simulink model "mcb_c2000_open_loop_control_host_model"  (R2021b)
settings: Solver=FixedStepDiscrete  StartTime=0.0  StopTime=inf  RelTol=1e-3  EnableMultiTasking=on
InitFcn:
  | if( strcmp(get_param([gcs '/Serial Communication/HW_Selected'], 'Value'), '0'))
  |       set_param([gcs '/Host Serial Setup'], 'baudRateA', '1.5e6');
  | elseif( strcmp(get_param([gcs '/Serial Communication/HW_Selected'], 'Value'), '1'))
  |       set_param([gcs '/Host Serial Setup'], 'baudRateA', '3.75e6');
  | elseif( strcmp(get_param([gcs '/Serial Communication/HW_Selected'], 'Value'), '2'))
  |       set_param([gcs '/Host Serial Setup'], 'baudRateA', '6.25e6');
  | end
values from neighbouring files (symbols this model uses):
  Ts = 5e-8    (= 5e-08)    [DCDC_Buck_Param.m]    (also in mcb_c2000_open_loop_control_data.m = T_pwm; mcb_c2000_pmsm_offset_data.m = T_pwm; mcb_pmsm_foc_dual_f28379d_data.m = 5e-05; mcb_pmsm_foc_dual_f28379d_datascript.m = 5e-05)
libraries: mcbhostblockslib x3, demo_controls x1
PreSaveFcn:
  | if( strcmp(get_param([gcs '/Serial Communication/HW_Selected'], 'Value'), '0'))
  |       set_param([gcs '/Host Serial Setup'], 'baudRateA', '1.5e6');
  | elseif( strcmp(get_param([gcs '/Serial Communication/HW_Selected'], 'Value'), '1'))
  |       set_param([gcs '/Host Serial Setup'], 'baudRateA', '3.75e6');
  | elseif( strcmp(get_param([gcs '/Serial Communication/HW_Selected'], 'Value'), '2'))
  |       set_param([gcs '/Host Serial Setup'], 'baudRateA', '6.25e6');
  | end
settings Model: Creator=The MathWorks, Inc.  LastModifiedBy=The MathWorks, Inc.
settings SolverCC: AlgebraicLoopSolver=TrustRegion
settings DataIOCC: LimitDataPoints=on  SaveFormat=Array  ReturnWorkspaceOutputs=off
settings OptimizationCC: LifeSpan=1  EfficientTunableParamExpr=on
settings DebuggingCC: UnderspecifiedInitializationDetection=Classic  MergeDetectMultiDrivingBlocksExec=none  SolverPrmCheckMsg=warning  ParameterPrecisionLossMsg=none  AllowSymbolicDim=off  PregeneratedLibrarySubsystemCodeDiagnostic=none  SFUnexpectedBacktrackingDiag=warning  SFNoUnconditionalDefaultTransitionDiag=warning  SFExecutionAtInitializationDiag=none  SFMachineParentedDataDiag=warning  ArithmeticOperatorsInVariantConditions=warning
settings HardwareCC: ProdBitPerPointer=32  ProdLargestAtomicFloat=None  ProdIntDivRoundTo=Undefined  ProdEndianess=Unspecified  ProdWordSize=32  ProdHWDeviceType=32-bit Generic
settings ModelReferenceCC: PropagateSignalLabelsOutOfModel=off
settings SFSimCC: SimUseLocalCustomCode=off  MATLABDynamicMemAlloc=off
settings RTWCC: Description=Real-Time Workshop Embedded Coder  SystemTargetFile=ert.tlc  TemplateMakefile=ert_default_tmf  GenerateReport=on  RTWUseLocalCustomCode=off  IncludeHyperlinkInReport=on  LaunchReport=on  GenerateTraceInfo=on  GenerateTraceReport=on  GenerateTraceReportSl=on  GenerateTraceReportSf=on  GenerateTraceReportEml=on
settings CodeAppCC: IgnoreCustomStorageClasses=off  StateflowObjectComments=on  InternalIdentifier=Classic
settings ERTTargetCC: MultiwordLength=2048  GenerateSampleERTMain=on  ERTCustomFileTemplate=example_file_process.tlc  ConvertIfToSwitch=off  SuppressUnreachableDefaultCases=off
settings ConfigComp: CovMetricSettings=dw  CovSaveCumulativeToWorkspaceVar=on  CovSaveSingleToWorkspaceVar=on  CovExternalEMLEnable=off  CovSFcnEnable=off

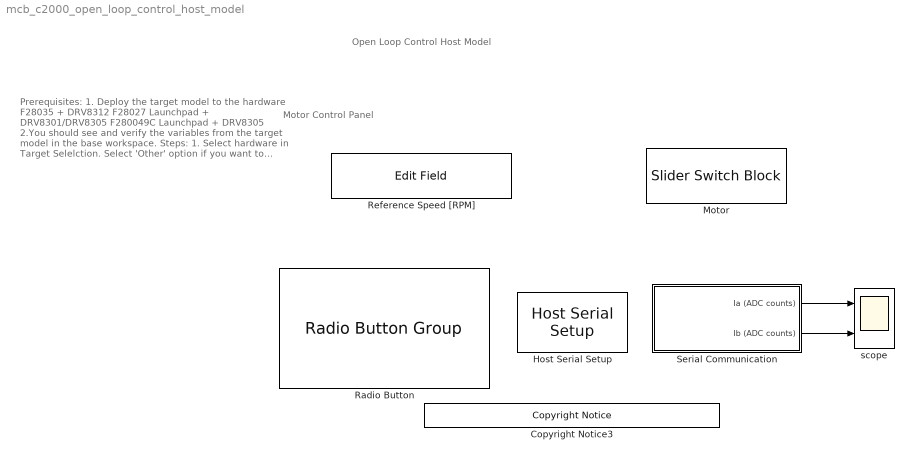
== system mcb_c2000_open_loop_control_host_model ==
  note: Open Loop Control Host Model
  note: Motor Control Panel
  note: Prerequisites:
      | 1. Deploy the target model to the hardware
      | F28035 + DRV8312
      | F28027 Launchpad + DRV8301/DRV8305
      | F280049C Launchpad + DRV8305
      | 2.You should see and verify the variables
      | from the target model in the base
      | workspace.
      |
      | Steps:
      | 1. Select hardware in Target Selelction.
      | Select 'Other' option if you want to manually set
      | the baud rate in 'Host Serial Setup' block.
      | 2. Select the serial port in ' Serial 1 ' tab of ' Host
      | Serial Setup ' block.
      | 3. Use ' Motor Start / Stop ' switch to control the
      | motor.
      | 4. Enter speed request in RPM using 'Reference
      | Speed' edit box. Limit the reference speed to
      | half of the rated speed.
      | 5. Observe the ADC counts for phase current
      | measurent in Scope.
  Copyright Notice3 : demo_controls/Copyright Notice  year=2021  prod=tic2000
      settings: SourceProductBaseCode=ME
  Host Serial Setup : mcbhostblockslib/Host Serial Setup  Priority=-99  comPortSer1='Please_select_a_port'  baudRateA=1.5e6  charLenA=8  stopBitA=1  parityA=none  timeoutA=2  ByteOrderA=LittleEndian  comPortSer2='Please_select_a_port'  baudRateB=115200  charLenB=8  stopBitB=1  parityB=none  timeoutB=1.0  ByteOrderB=LittleEndian  comPortSer3='Please_select_a_port'  baudRateC=115200  charLenC=8  stopBitC=1  parityC=none  timeoutC=1.0  ByteOrderC=LittleEndian  comPortSer4='Please_select_a_port'  baudRateD=115200  charLenD=8  stopBitD=1  parityD=none  timeoutD=1.0  ByteOrderD=LittleEndian
      settings: SourceProductBaseCode=MT
  Motor : SliderSwitchBlock  LabelPosition=Hide
      settings: Values={{'Stop', 'Start'}, [0 1]}
  Radio Button : RadioButtonGroup  LabelPosition=Hide  SelectedLabel=TI F28035  ButtonGroupName=Target Selection
      settings: Values={{'TI F28035', 'TI F28027', 'TI F280049C', 'Other'}, [0 1 2 3]}
  Reference Speed [RPM] : EditField  LabelPosition=Hide  ShowInitialText=on  Alignment=Center
  Serial Communication : Subsystem
  scope : Scope  NumInputPorts=2
  wires:
  Serial Communication/1(Ia (ADC counts)) -> scope/1
  Serial Communication/2(Ib (ADC counts)) -> scope/2

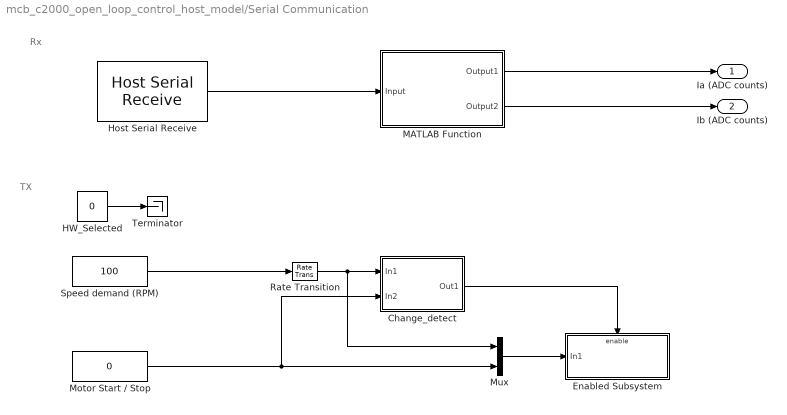
== system mcb_c2000_open_loop_control_host_model/Serial Communication ==
  note: TX
  note: Rx
  Change_detect : Subsystem
  Enabled Subsystem : Subsystem  TreatAsAtomicUnit=on
  HW_Selected : Constant  Value=0  OutDataTypeStr=uint8
  Host Serial Receive : mcbhostblockslib/Host Serial Receive  serialCon=Serial 1  dataHead='SS'  dataTail='EE'  dataType=uint16  dataDim=[600 2]  initValue=0  errOption=Output the last received value  errValue=0  sampleTime=600 * Ts  outputStatus=off  blockingMode=on
      settings: SourceProductBaseCode=MT
  MATLAB Function : MATLAB Function  TreatAsAtomicUnit=on
  Motor Start / Stop : Constant  Value=0  VectorParams1D=off  OutDataTypeStr=single  SampleTime=0.03
  Mux : Mux  Inputs=2
  Rate Transition : RateTransition  OutPortSampleTime=0.03
  Speed demand (RPM) : Constant  Value=100  VectorParams1D=off  OutDataTypeStr=single  SampleTime=0.03
  Terminator : Terminator
  Ia (ADC counts) : Outport
  Ib (ADC counts) : Outport  Port=2
  wires:
  Host Serial Receive/1 -> MATLAB Function/1(Input)
  MATLAB Function/2(Output2) -> Ib (ADC counts)/1
  MATLAB Function/1(Output1) -> Ia (ADC counts)/1
  HW_Selected/1 -> Terminator/1
  Change_detect/1(Out1) -> Enabled Subsystem/Enable
  Mux/1 -> Enabled Subsystem/1(In1)
  Rate Transition/1 -> Change_detect/1(In1), Mux/1
  Motor Start / Stop/1 -> Change_detect/2(In2), Mux/2
  Speed demand (RPM)/1 -> Rate Transition/1

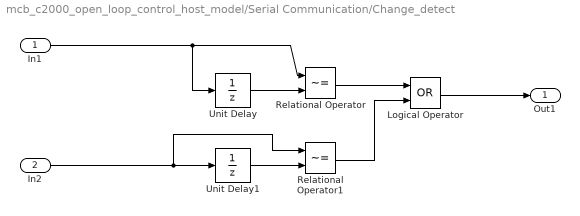
== system mcb_c2000_open_loop_control_host_model/Serial Communication/Change_detect ==
  In1 : Inport
  In2 : Inport  Port=2
  Logical Operator : Logic  Operator=OR  AllPortsSameDT=off  OutDataTypeStr=boolean
  Relational Operator : RelationalOperator  Operator=~=  OutDataTypeStr=boolean  RndMeth=Nearest
  Relational Operator1 : RelationalOperator  Operator=~=  OutDataTypeStr=boolean  RndMeth=Nearest
  Unit Delay : UnitDelay  InitialCondition=0.5  SampleTime=-1  HasFrameUpgradeWarning=on
  Unit Delay1 : UnitDelay  SampleTime=-1  HasFrameUpgradeWarning=on
  Out1 : Outport  VectorParamsAs1DForOutWhenUnconnected=off
  wires:
  In2/1 -> Relational Operator1/1, Unit Delay1/1
  Relational Operator1/1 -> Logical Operator/2
  Unit Delay1/1 -> Relational Operator1/2
  Unit Delay/1 -> Relational Operator/2
  In1/1 -> Unit Delay/1, Relational Operator/1
  Relational Operator/1 -> Logical Operator/1
  Logical Operator/1 -> Out1/1

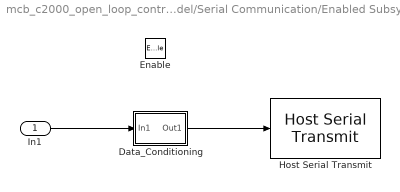
== system mcb_c2000_open_loop_control_host_model/Serial Communication/Enabled Subsystem ==
  In1 : Inport
  Enable : EnablePort
  Data_Conditioning : Subsystem
  Host Serial Transmit : mcbhostblockslib/Host Serial Transmit  serialCon=Serial 1  header=''  tail=''  enableBlockingMode=off
      settings: SourceProductBaseCode=MT
  wires:
  In1/1 -> Data_Conditioning/1(In1)
  Data_Conditioning/1(Out1) -> Host Serial Transmit/1

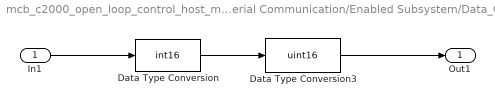
== system mcb_c2000_open_loop_control_host_model/Serial Communication/Enabled Subsystem/Data_Conditioning ==
  In1 : Inport
  Data Type Conversion : DataTypeConversion  OutDataTypeStr=int16  RndMeth=Simplest
  Data Type Conversion3 : DataTypeConversion  OutDataTypeStr=uint16  ConvertRealWorld=Stored Integer (SI)  RndMeth=Simplest
  Out1 : Outport  VectorParamsAs1DForOutWhenUnconnected=off
  wires:
  In1/1 -> Data Type Conversion/1
  Data Type Conversion3/1 -> Out1/1
  Data Type Conversion/1 -> Data Type Conversion3/1

== matlab function mcb_c2000_open_loop_control_host_model/Serial Communication/MATLAB Function ==
  data: Output1 output; Output2 output; Input input
function [ Output1, Output2] = unBuf(Input)

Output1= Input(:, 1);
Output2 = Input(:, 2);
end
